simulink model "controlallocationblock"  (R2015b)
settings: Solver=VariableStepAuto  StartTime=0.0  StopTime=1  RelTol=1e-3
libraries: dspmtrx3 x3
settings Model: Creator=ADMIN  LastModifiedBy=ADMIN

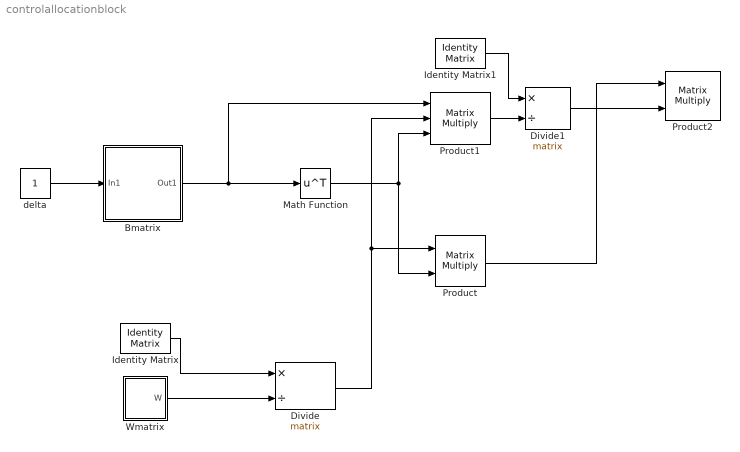
== system controlallocationblock ==
  "Bmatrix " : Subsystem
  Divide : Product  Inputs=*/  Multiplication=Matrix(*)
  Divide1 : Product  Inputs=*/  Multiplication=Matrix(*)
  Identity Matrix : dspmtrx3/Identity Matrix  Inherit=off  N=4  Ts=1  dataType=double  isSigned=on  wordLen=16  udDataType=sfix(16)  fracBitsMode=Best precision  numFracBits=15  OutDataTypeStr=double  LastOutDataTypeStr=double
  Identity Matrix1 : dspmtrx3/Identity Matrix  Inherit=off  N=2  Ts=1  dataType=double  isSigned=on  wordLen=16  udDataType=sfix(16)  fracBitsMode=Best precision  numFracBits=15  OutDataTypeStr=double  LastOutDataTypeStr=double
  Math Function : Math  Operator=transpose  SaturateOnIntegerOverflow=on
  Product : Product  Multiplication=Matrix(*)
  Product1 : Product  Inputs=3  Multiplication=Matrix(*)
  Product2 : Product  Multiplication=Matrix(*)
  Wmatrix : Subsystem
  delta : Constant
  wires:
  delta/1 -> "Bmatrix "/1(In1)
  "Bmatrix "/1(Out1) -> Product1/1, Math Function/1
  Identity Matrix/1 -> Divide/1
  Wmatrix/1(W) -> Divide/2
  Divide/1 -> Product1/2, Product/1
  Math Function/1 -> Product1/3, Product/2
  Product/1 -> Product2/1
  Identity Matrix1/1 -> Divide1/1
  Product1/1 -> Divide1/2
  Divide1/1 -> Product2/2

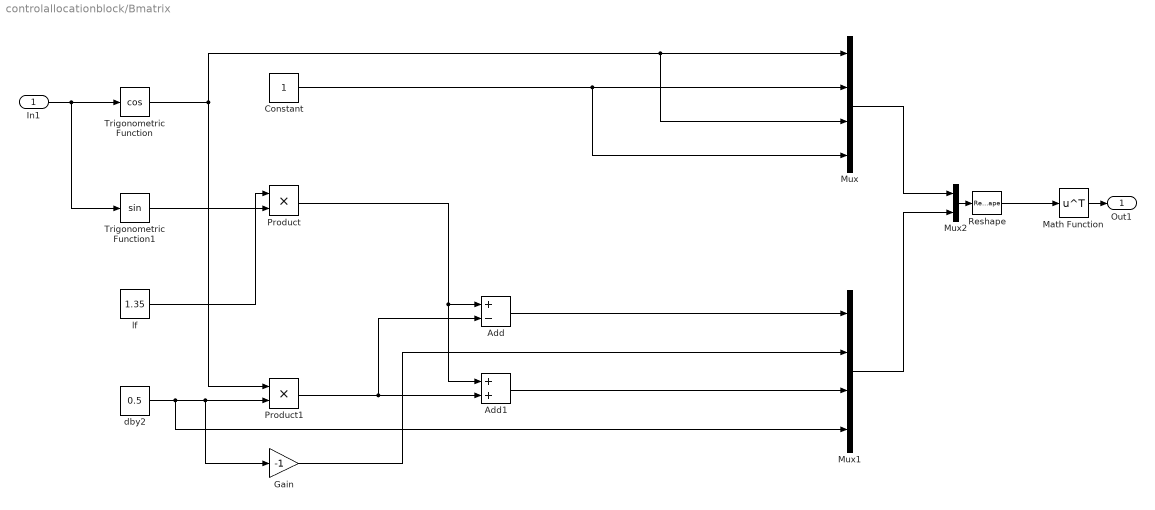
== system controlallocationblock/Bmatrix  ==
  In1 : Inport
  Add : Sum  Inputs=+-
  Add1 : Sum
  Constant : Constant
  Gain : Gain  Gain=-1
  Math Function : Math  Operator=transpose  SaturateOnIntegerOverflow=on
  Mux : Mux
  Mux1 : Mux
  Mux2 : Mux  Inputs=2
  Product : Product
  Product1 : Product
  Reshape : Reshape  OutputDimensionality=Customize  OutputDimensions=[4,2]
  Trigonometric Function : Trigonometry  Operator=cos
  Trigonometric Function1 : Trigonometry
  dby2 : Constant  Value=0.5
  lf : Constant  Value=1.35
  Out1 : Outport
  wires:
  Mux2/1 -> Reshape/1
  Product1/1 -> Add/2, Add1/2
  Reshape/1 -> Math Function/1
  Gain/1 -> Mux1/2
  Mux/1 -> Mux2/1
  Add/1 -> Mux1/1
  Add1/1 -> Mux1/3
  Trigonometric Function1/1 -> Product/2
  Trigonometric Function/1 -> Product1/1, Mux/3, Mux/1
  Constant/1 -> Mux/2, Mux/4
  In1/1 -> Trigonometric Function1/1, Trigonometric Function/1
  Product/1 -> Add1/1, Add/1
  dby2/1 -> Mux1/4, Gain/1, Product1/2
  lf/1 -> Product/1
  Mux1/1 -> Mux2/2
  Math Function/1 -> Out1/1

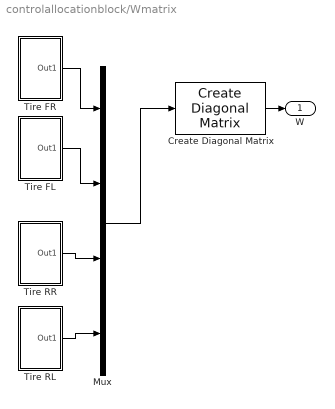
== system controlallocationblock/Wmatrix ==
  Create Diagonal Matrix : dspmtrx3/Create Diagonal Matrix
  Mux : Mux
  Tire FL : Subsystem
  Tire FR : Subsystem
  Tire RL : Subsystem
  Tire RR : Subsystem
  W : Outport
  wires:
  Tire RR/1(Out1) -> Mux/3
  Tire RL/1(Out1) -> Mux/4
  Mux/1 -> Create Diagonal Matrix/1
  Tire FL/1(Out1) -> Mux/2
  Tire FR/1(Out1) -> Mux/1
  Create Diagonal Matrix/1 -> W/1

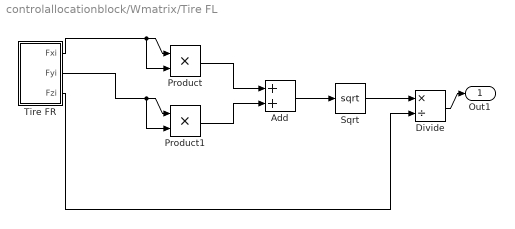
== system controlallocationblock/Wmatrix/Tire FL ==
  Add : Sum
  Divide : Product  Inputs=*/
  Product : Product
  Product1 : Product
  Sqrt : Sqrt  SaturateOnIntegerOverflow=on
  Tire FR : Subsystem
  Out1 : Outport
  wires:
  Add/1 -> Sqrt/1
  Product1/1 -> Add/2
  Product/1 -> Add/1
  Tire FR/3(Fzi) -> Divide/2
  Divide/1 -> Out1/1
  Sqrt/1 -> Divide/1
  Tire FR/2(Fyi) -> Product1/2, Product1/1
  Tire FR/1(Fxi) -> Product/2, Product/1

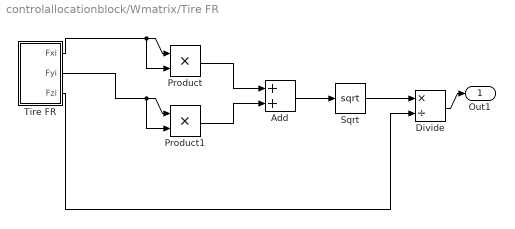
== system controlallocationblock/Wmatrix/Tire FR ==
  Add : Sum
  Divide : Product  Inputs=*/
  Product : Product
  Product1 : Product
  Sqrt : Sqrt  SaturateOnIntegerOverflow=on
  Tire FR : Subsystem
  Out1 : Outport
  wires:
  Add/1 -> Sqrt/1
  Product1/1 -> Add/2
  Product/1 -> Add/1
  Tire FR/3(Fzi) -> Divide/2
  Divide/1 -> Out1/1
  Sqrt/1 -> Divide/1
  Tire FR/2(Fyi) -> Product1/2, Product1/1
  Tire FR/1(Fxi) -> Product/2, Product/1

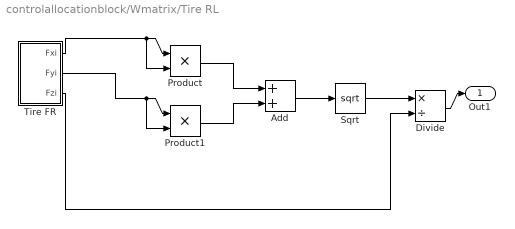
== system controlallocationblock/Wmatrix/Tire RL ==
  Add : Sum
  Divide : Product  Inputs=*/
  Product : Product
  Product1 : Product
  Sqrt : Sqrt  SaturateOnIntegerOverflow=on
  Tire FR : Subsystem
  Out1 : Outport
  wires:
  Add/1 -> Sqrt/1
  Product1/1 -> Add/2
  Product/1 -> Add/1
  Tire FR/3(Fzi) -> Divide/2
  Divide/1 -> Out1/1
  Sqrt/1 -> Divide/1
  Tire FR/2(Fyi) -> Product1/2, Product1/1
  Tire FR/1(Fxi) -> Product/2, Product/1

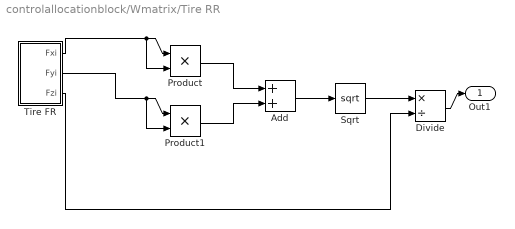
== system controlallocationblock/Wmatrix/Tire RR ==
  Add : Sum
  Divide : Product  Inputs=*/
  Product : Product
  Product1 : Product
  Sqrt : Sqrt  SaturateOnIntegerOverflow=on
  Tire FR : Subsystem
  Out1 : Outport
  wires:
  Add/1 -> Sqrt/1
  Product1/1 -> Add/2
  Product/1 -> Add/1
  Tire FR/3(Fzi) -> Divide/2
  Divide/1 -> Out1/1
  Sqrt/1 -> Divide/1
  Tire FR/2(Fyi) -> Product1/2, Product1/1
  Tire FR/1(Fxi) -> Product/2, Product/1

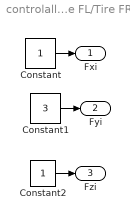
== system controlallocationblock/Wmatrix/Tire FL/Tire FR ==
  Constant : Constant
  Constant1 : Constant  Value=3
  Constant2 : Constant
  Fxi : Outport
  Fyi : Outport  Port=2
  Fzi : Outport  Port=3
  wires:
  Constant2/1 -> Fzi/1
  Constant/1 -> Fxi/1
  Constant1/1 -> Fyi/1

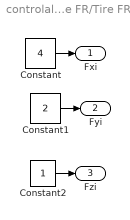
== system controlallocationblock/Wmatrix/Tire FR/Tire FR ==
  Constant : Constant  Value=4
  Constant1 : Constant  Value=2
  Constant2 : Constant
  Fxi : Outport
  Fyi : Outport  Port=2
  Fzi : Outport  Port=3
  wires:
  Constant2/1 -> Fzi/1
  Constant/1 -> Fxi/1
  Constant1/1 -> Fyi/1

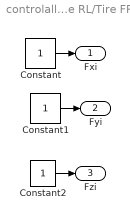
== system controlallocationblock/Wmatrix/Tire RL/Tire FR ==
  Constant : Constant
  Constant1 : Constant
  Constant2 : Constant
  Fxi : Outport
  Fyi : Outport  Port=2
  Fzi : Outport  Port=3
  wires:
  Constant2/1 -> Fzi/1
  Constant/1 -> Fxi/1
  Constant1/1 -> Fyi/1

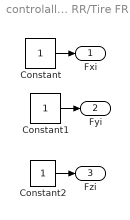
== system controlallocationblock/Wmatrix/Tire RR/Tire FR ==
  Constant : Constant
  Constant1 : Constant
  Constant2 : Constant
  Fxi : Outport
  Fyi : Outport  Port=2
  Fzi : Outport  Port=3
  wires:
  Constant2/1 -> Fzi/1
  Constant/1 -> Fxi/1
  Constant1/1 -> Fyi/1
